simulink model "HVDC_MMC1_EMT"  (R2023b)
settings: Solver=ode23tb  StartTime=0.0  StopTime=10  MaxStep=Ts  RelTol=1e-3  EnableMultiTasking=on
PreLoadFcn:
  | HVDC_MMC_param
StartFcn:
  | tic
StopFcn:
  | toc
values from neighbouring files (symbols this model uses):
  acdcV = 1/(Vnom_dc/2*sqrt(3)/sqrt(2)/Vnom_sec)    [HVDC_MMC_param.m]
  C_PM = 1.758e-3    (= 0.001758)    [HVDC_MMC_param.m]
  Carm = 1.0*C_pm/n    (= 0.0002096)    [B2B_HVDC_MMC_Calc.m]    (also in HVDC_MMC_param.m = 4.88333333333e-05)
  DC_cable_C_shunt = 0.1e-6    (= 1e-07)    [HVDC_MMC_param.m]
  DC_cable_R_shunt = 1000    [HVDC_MMC_param.m]
  DCM = 1    [HVDC_MMC_param.m]
  Fn_filter = 1000    [B2B_HVDC_MMC_Calc.m]    (also in HVDC_MMC_param.m)
  Fnom = 50    [HVDC_MMC_param.m]
  HRM = 2    [HVDC_MMC_param.m]
  HrmOrd = N    (= 2)    [B2B_HVDC_MMC_Calc.m]    (also in HVDC_MMC_param.m)
  Ib_ac = (2/3)*Pnom/Vb_ac    [HVDC_MMC_param.m]
  Ib_dc = Pnom/Vb_dc    (= 1501.5015015)    [HVDC_MMC_param.m]
  Ki_CCSC = 50    [HVDC_MMC_param.m]
  Ki_Ireg = 6    [HVDC_MMC_param.m]
  Ki_Preg = 1.0    (= 1)    [HVDC_MMC_param.m]
  Ki_Qreg = 1.0    (= 1)    [HVDC_MMC_param.m]
  Ki_VDCreg = 100    [HVDC_MMC_param.m]
  Kp_CCSC = 0.8    [HVDC_MMC_param.m]
  Kp_Ireg = 0.6    [HVDC_MMC_param.m]
  Kp_Preg = 0.5/3    (= 0.166666666667)    [HVDC_MMC_param.m]
  Kp_Qreg = 0.5/3    (= 0.166666666667)    [HVDC_MMC_param.m]
  Kp_VDCreg = 4    [HVDC_MMC_param.m]
  L_cable = 15e-3    (= 0.015)    [HVDC_MMC_param.m]
  Larm = Larm_pu*(Zb_ac/w)    [HVDC_MMC_param.m]
  Lff = Larm_pu/2+Lxfo    (= 0.195)    [HVDC_MMC_param.m]
  Limits_Ireg = [ 2.0  -2.0]    [HVDC_MMC_param.m]
  Limits_Preg = [ 1.2, 0.8 ]    [HVDC_MMC_param.m]
  Limits_Qreg = [ 0.25, -0.25 ]    [HVDC_MMC_param.m]
  Limits_VDCreg = [ 2.0  -2.0]    [HVDC_MMC_param.m]
  Lxfo = 0.12    [HVDC_MMC_param.m]
  Pac = 0.9    [HVDC_MMC_param.m]
  Pnom = 1000e6    (= 1000000000)    [HVDC_MMC_param.m]
  Qac = 0.2    [HVDC_MMC_param.m]
  QCM = 0    [HVDC_MMC_param.m]
  R_cable = 0.5    [HVDC_MMC_param.m]
  Rarm = Rarm_pu*Zb_ac    [HVDC_MMC_param.m]
  Rff = Rarm_pu/2+Rxfo    (= 0.00375)    [HVDC_MMC_param.m]
  Rxfo = 0.003    [HVDC_MMC_param.m]
  Slope_Pref = 0.5    [HVDC_MMC_param.m]
  Slope_Qref = 0.5    [HVDC_MMC_param.m]
  Slope_Vdc_ref = Vnom_dc/5    (= 133200)    [HVDC_MMC_param.m]
  Tbrk1_On = 0.1    [HVDC_MMC_param.m]
  Tbrk2_On = 1.0    (= 1)    [HVDC_MMC_param.m]
  Tdeblock = 1.5    [HVDC_MMC_param.m]
  Tfault = 9999    [HVDC_MMC_param.m]
  Ton_Converter2 = 3    [HVDC_MMC_param.m]
  Ton_PQreg = 2    [HVDC_MMC_param.m]
  Ton_VDCreg = 1.5    [HVDC_MMC_param.m]
  Ts = Ts_Power    (= 5e-05)    [B2B_HVDC_MMC_Calc.m]    (also in HVDC_MMC_param.m)
  Ts_Control = Ts_Power    (= 5e-05)    [B2B_HVDC_MMC_Calc.m]    (also in HVDC_MMC_param.m)
  Ts_DQN = MultTs*Ts_Power    (= 5e-05)    [B2B_HVDC_MMC_Calc.m]    (also in HVDC_MMC_param.m)
  Ts_EMT = Ts    (= 5e-05)    [HVDC_MMC_param.m]
  Ts_Power = 1*50e-6    (= 5e-05)    [B2B_HVDC_MMC_Calc.m]    (also in HVDC_MMC_param.m)
  Vb_ac = sqrt(2/3)*Vnom_sec    [HVDC_MMC_param.m]
  Vb_dc = Vnom_dc    (= 666000)    [HVDC_MMC_param.m]
  Vc0_PM = 0    [HVDC_MMC_param.m]
  Vnom_dc = 2*Vnom_sec    (= 666000)    [HVDC_MMC_param.m]
  Vnom_prim = 333e3    (= 333000)    [HVDC_MMC_param.m]
  Vnom_sec = 333e3    (= 333000)    [HVDC_MMC_param.m]
  w = 2*pi*f    (= 314.159265359)    [B2B_HVDC_MMC_Calc.m]    (also in HVDC_MMC_param.m)
  Ws = 2*pi*Fnom    (= 314.159265359)    [HVDC_MMC_param.m]
  Zb_ac = Vb_ac/Ib_ac    [HVDC_MMC_param.m]
  Zeta_filter = 1    [B2B_HVDC_MMC_Calc.m]    (also in HVDC_MMC_param.m)
undefined symbols (not defined in the file or in its folder): DCss, DiscIntNeverNeededParam, gcbh, MT, sps_rtmsupport
libraries: DQN_Lib x37, simulink x35, spsCurrentMeasurementLib x24, powerlib_extras x21, slpidlib x14, spsSecondOrderFilterLib x14, spsVoltageMeasurementLib x10, spsSeriesRLCBranchLib x10, spsControlledVoltageSourceLib x9, spsHalfBridgeMMCmodel x7, spsGroundLib x4, spsParallelRLCBranchLib x4
(part 5 of 9)

== system HVDC_MMC1_EMT/MMC/RHB ==
  Uref : Inport  SampleTime=Ts
  Controlled Voltage Source : spsControlledVoltageSourceLib/Controlled Voltage Source  Initialize=on  Source_Type=AC  Amplitude=0  Phase=0  Frequency=0  Measurements=None
  Controlled Voltage Source2 : spsControlledVoltageSourceLib/Controlled Voltage Source  Initialize=on  Source_Type=AC  Amplitude=0  Phase=0  Frequency=0  Measurements=None
  Current Measurement : spsCurrentMeasurementLib/Current Measurement  PhasorSimulation=off  OutputType=Complex  PSBequivalent=0
  Current Measurement1 : spsCurrentMeasurementLib/Current Measurement  PhasorSimulation=off  OutputType=Complex  PSBequivalent=0
  Demux : Demux  Outputs=2
  Diode : spsDiodeLib/Diode  Ron=Ron_Diode  Lon=0  Vf=Vf_Diode  IC=0  UseSnubber=0  Rs=Rs_Diode  Cs=Cs_Diode  Measurements=off
  Diode1 : spsDiodeLib/Diode  Ron=Ron_Diode  Lon=0  Vf=Vf_Diode  IC=0  UseSnubber=0  Rs=Rs_Diode  Cs=Cs_Diode  Measurements=off
  Discrete-Time Integrator : DiscreteIntegrator  IntegratorMethod=Integration: Trapezoidal  gainval=1  InitialCondition=Vc_Initial  SampleTime=Ts  UpperSaturationLimit=5000  LowerSaturationLimit=500  ICPrevOutput=DiscIntNeverNeededParam  ICPrevScaledInput=DiscIntNeverNeededParam
  Gain : Gain  Gain=1/(C*n)
  Gain2 : Gain  Gain=2
  Mux : Mux  Inputs=2
  Mux1 : Mux  Inputs=2
  Product1 : Product
  Product2 : Product
  Sum1 : Sum  Inputs=1  InputSameDT=on  SaturateOnIntegerOverflow=on  OutDataTypeStr=Inherit: Same as first input
  Sum2 : Sum  Inputs=+-  InputSameDT=on  SaturateOnIntegerOverflow=on  OutDataTypeStr=Inherit: Same as first input
  Unit Delay1 : UnitDelay  SampleTime=Ts  HasFrameUpgradeWarning=on
  Unit Delay3 : UnitDelay  InitialCondition=Vc_Initial  SampleTime=Ts  HasFrameUpgradeWarning=on
  Unit Delay4 : UnitDelay  InitialCondition=Vc_Initial  SampleTime=Ts  HasFrameUpgradeWarning=on
  1 : PMIOPort  Side=Right
  2 : PMIOPort  Port=2  Side=Right
  wires:
  Unit Delay4/1 -> Gain2/1, Unit Delay3/1
  Gain2/1 -> Sum2/1
  Demux/2 -> Controlled Voltage Source2/1
  Sum1/1 -> Gain/1
  Product2/1 -> Demux/1
  Unit Delay3/1 -> Sum2/2
  Mux/1 -> Unit Delay1/1
  Unit Delay1/1 -> Product1/2
  Discrete-Time Integrator/1 -> Unit Delay4/1
  [Icap] -> Mux/2
  Current Measurement1/1 -> [Icap]
  Product1/1 -> Sum1/1
  Current Measurement/1 -> [Imod]
  Mux1/1 -> Product1/1, Product2/1
  Demux/1 -> Controlled Voltage Source/1
  Gain/1 -> Discrete-Time Integrator/1
  Sum2/1 -> Product2/2
  [Imod] -> Mux/1
  Uref/1 -> Mux1/2, Mux1/1
  connections:
  Current Measurement/RConn1 -- Diode1/RConn1 -- Diode/LConn1
  2/RConn1 -- Diode1/LConn1 -- Controlled Voltage Source2/LConn1
  Controlled Voltage Source/RConn1 -- 1/RConn1
  Current Measurement1/RConn1 -- Controlled Voltage Source2/RConn1
  Current Measurement/LConn1 -- Controlled Voltage Source/LConn1
  Diode/RConn1 -- Current Measurement1/LConn1

== system HVDC_MMC1_EMT/MMC/Subsystem ==
  Current Measurement1 : spsCurrentMeasurementLib/Current Measurement  PhasorSimulation=off  OutputType=Complex  PSBequivalent=0
  Voltage Measurement : spsVoltageMeasurementLib/Voltage Measurement  PhasorSimulation=off  OutputType=Complex  PSBequivalent=0
  I1 : PMIOPort  Side=Left
  I2 : PMIOPort  Port=2  Side=Left
  O1 : PMIOPort  Port=3  Side=Right
  O2 : PMIOPort  Port=4  Side=Right
  tag scope: I_Ap=global, V12_Ap=global
  wires:
  Current Measurement1/1 -> [I_Ap]
  Voltage Measurement/1 -> [V12_Ap]
  connections:
  Current Measurement1/RConn1 -- Voltage Measurement/LConn1 -- I1/RConn1
  Current Measurement1/LConn1 -- O1/RConn1
  I2/RConn1 -- Voltage Measurement/LConn2 -- O2/RConn1

== system HVDC_MMC1_EMT/MMC/Subsystem1 ==
  Current Measurement1 : spsCurrentMeasurementLib/Current Measurement  PhasorSimulation=off  OutputType=Complex  PSBequivalent=0
  Voltage Measurement : spsVoltageMeasurementLib/Voltage Measurement  PhasorSimulation=off  OutputType=Complex  PSBequivalent=0
  I1 : PMIOPort  Side=Left
  I2 : PMIOPort  Port=2  Side=Left
  O1 : PMIOPort  Port=3  Side=Right
  O2 : PMIOPort  Port=4  Side=Right
  tag scope: I_Am=global, V12_Am=global
  wires:
  Voltage Measurement/1 -> [V12_Am]
  Current Measurement1/1 -> [I_Am]
  connections:
  Voltage Measurement/LConn2 -- O2/RConn1 -- I2/RConn1
  Current Measurement1/LConn1 -- O1/RConn1
  Voltage Measurement/LConn1 -- Current Measurement1/RConn1 -- I1/RConn1

== system HVDC_MMC1_EMT/MMC/Subsystem2 ==
  Current Measurement1 : spsCurrentMeasurementLib/Current Measurement  PhasorSimulation=off  OutputType=Complex  PSBequivalent=0
  Voltage Measurement : spsVoltageMeasurementLib/Voltage Measurement  PhasorSimulation=off  OutputType=Complex  PSBequivalent=0
  I1 : PMIOPort  Side=Left
  I2 : PMIOPort  Port=2  Side=Left
  O1 : PMIOPort  Port=3  Side=Right
  O2 : PMIOPort  Port=4  Side=Right
  tag scope: I_Bp=global, V12_Bp=global
  wires:
  Voltage Measurement/1 -> [V12_Bp]
  Current Measurement1/1 -> [I_Bp]
  connections:
  Voltage Measurement/LConn2 -- O2/RConn1 -- I2/RConn1
  Current Measurement1/LConn1 -- O1/RConn1
  Voltage Measurement/LConn1 -- Current Measurement1/RConn1 -- I1/RConn1

== system HVDC_MMC1_EMT/MMC/Subsystem3 ==
  Current Measurement1 : spsCurrentMeasurementLib/Current Measurement  PhasorSimulation=off  OutputType=Complex  PSBequivalent=0
  Voltage Measurement : spsVoltageMeasurementLib/Voltage Measurement  PhasorSimulation=off  OutputType=Complex  PSBequivalent=0
  I1 : PMIOPort  Side=Left
  I2 : PMIOPort  Port=2  Side=Left
  O1 : PMIOPort  Port=3  Side=Right
  O2 : PMIOPort  Port=4  Side=Right
  tag scope: I_Bm=global, V12_Bm=global
  wires:
  Current Measurement1/1 -> [I_Bm]
  Voltage Measurement/1 -> [V12_Bm]
  connections:
  I1/RConn1 -- Current Measurement1/RConn1 -- Voltage Measurement/LConn1
  Current Measurement1/LConn1 -- O1/RConn1
  I2/RConn1 -- O2/RConn1 -- Voltage Measurement/LConn2

== system HVDC_MMC1_EMT/MMC/Subsystem4 ==
  Current Measurement1 : spsCurrentMeasurementLib/Current Measurement  PhasorSimulation=off  OutputType=Complex  PSBequivalent=0
  Voltage Measurement : spsVoltageMeasurementLib/Voltage Measurement  PhasorSimulation=off  OutputType=Complex  PSBequivalent=0
  I1 : PMIOPort  Side=Left
  I2 : PMIOPort  Port=2  Side=Left
  O1 : PMIOPort  Port=3  Side=Right
  O2 : PMIOPort  Port=4  Side=Right
  tag scope: I_Cp=global, V12_Cp=global
  wires:
  Current Measurement1/1 -> [I_Cp]
  Voltage Measurement/1 -> [V12_Cp]
  connections:
  I1/RConn1 -- Current Measurement1/RConn1 -- Voltage Measurement/LConn1
  Current Measurement1/LConn1 -- O1/RConn1
  I2/RConn1 -- O2/RConn1 -- Voltage Measurement/LConn2

== system HVDC_MMC1_EMT/MMC/Subsystem5 ==
  Current Measurement1 : spsCurrentMeasurementLib/Current Measurement  PhasorSimulation=off  OutputType=Complex  PSBequivalent=0
  Voltage Measurement : spsVoltageMeasurementLib/Voltage Measurement  PhasorSimulation=off  OutputType=Complex  PSBequivalent=0
  I1 : PMIOPort  Side=Left
  I2 : PMIOPort  Port=2  Side=Left
  O1 : PMIOPort  Port=3  Side=Right
  O2 : PMIOPort  Port=4  Side=Right
  tag scope: I_Cm=global, V12_Cm=global
  wires:
  Voltage Measurement/1 -> [V12_Cm]
  Current Measurement1/1 -> [I_Cm]
  connections:
  Voltage Measurement/LConn2 -- O2/RConn1 -- I2/RConn1
  Current Measurement1/LConn1 -- O1/RConn1
  Voltage Measurement/LConn1 -- Current Measurement1/RConn1 -- I1/RConn1

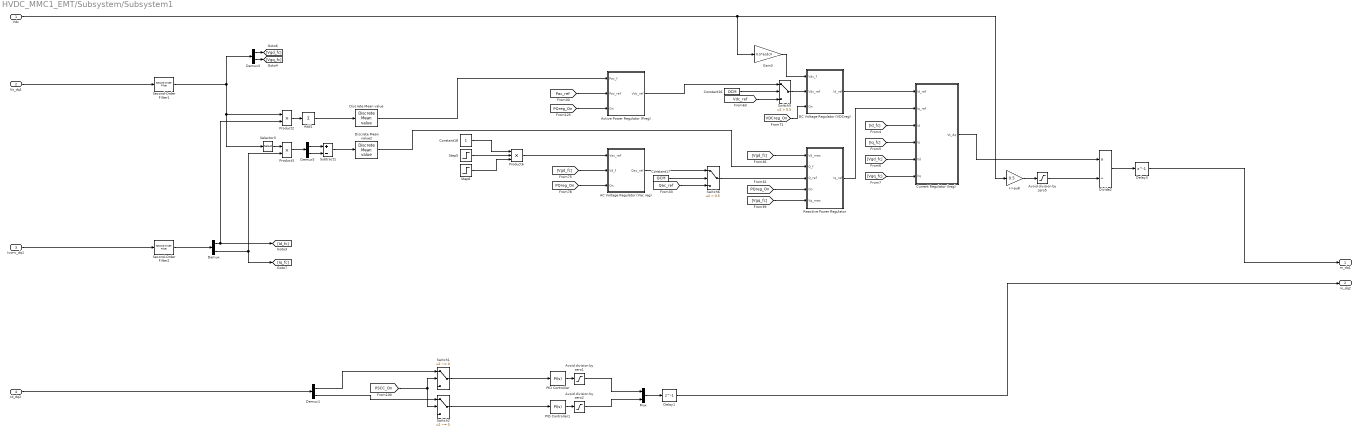
== system HVDC_MMC1_EMT/Subsystem/Subsystem1 ==
  Vdc : Inport
  Vs_dq1 : Inport  Port=2
  Iconv_dq1 : Inport  Port=3
  Id_dq2 : Inport  Port=4
  AC Voltage Regulator (Vac reg) : Subsystem
  Active Power Regulator (Preg) : Subsystem
  Add1 : Sum  Inputs=1
  Avoid division by zero1 : Saturate  UpperLimit=2  LowerLimit=-2
  Avoid division by zero2 : Saturate  UpperLimit=2  LowerLimit=-2
  Avoid division by zero5 : Saturate  UpperLimit=10*acdcV  LowerLimit=0.5/acdcV  ZeroCross=off
  Constant16 : Constant  Value=DCM
  Constant17 : Constant  Value=QCM
  Constant18 : Constant
  Current Regulator (Ireg) : Subsystem
  DC Voltage Regulator (VDCreg) : Subsystem
  Delay1 : Delay  DelayLength=1
  Delay3 : Delay  DelayLength=1
  Demux{,1,3,5} (4 alike) : Demux  Outputs=2
  Discrete Mean value : powerlib_extras/Discrete Measurements/Discrete  Mean value  Freq=Fnom  Vinit=0  Ts=Ts
  Discrete Mean value2 : powerlib_extras/Discrete Measurements/Discrete  Mean value  Freq=Fnom  Vinit=0  Ts=Ts
  Divide2 : Product  Inputs=*/
  Gain3 : Gain  Gain=0.5*acdcV
  I->pu8 : Gain  Gain=0.5  SaturateOnIntegerOverflow=on  OutDataTypeStr=Inherit: Same as input  ParamDataTypeStr=Inherit: Same as input
  Mux : Mux  Inputs=2
  PID Controller : slpidlib/PID Controller  Controller=PI  Form=Parallel  TimeDomain=Continuous-time  UseExternalTs=off  SampleTime=-1  IntegratorMethod=Forward Euler  FilterMethod=Forward Euler  ControllerParametersSource=internal  P=Kp_CCSC  I=Ki_CCSC  UseKiTs=off  D=0  N=100  UseFilter=on  TunerSelectOption=Transfer Function Based (PID Tuner App)  InitialConditionSource=internal  InitialConditionForIntegrator=0  InitialConditionForFilter=0  DifferentiatorICPrevScaledInput=0  ExternalReset=none  TrackingMode=off  Kt=1  LimitOutput=off  SatLimitsSource=internal  UpperSaturationLimit=inf  LowerSaturationLimit=-inf  LinearizeAsGain=on  AntiWindupMode=none  Kb=1  LimitIntegrator=off  UpperIntegratorSaturationLimit=inf  LowerIntegratorSaturationLimit=-inf  POutMin=[]  POutMax=[]  IOutMin=[]  IOutMax=[]  DOutMin=[]  DOutMax=[]  NOutMin=[]  NOutMax=[]  SumOutMin=[]  SumOutMax=[]  SaturationOutMin=[]  SaturationOutMax=[]  PParamMin=[]  PParamMax=[]  IParamMin=[]  IParamMax=[]  DParamMin=[]  DParamMax=[]  NParamMin=[]  NParamMax=[]  KbParamMin=[]  KbParamMax=[]  KtParamMin=[]  KtParamMax=[]  KbOutMin=[]  KbOutMax=[]  KtOutMin=[]  KtOutMax=[]  IntegratorOutMin=[]  IntegratorOutMax=[]  FilterOutMin=[]  FilterOutMax=[]  SumI1OutMin=[]  SumI1OutMax=[]  SumI2OutMin=[]  SumI2OutMax=[]  SumI3OutMin=[]  SumI3OutMax=[]  SumI4OutMin=[]  SumI4OutMax=[]  SumDOutMin=[]  SumDOutMax=[]  DifferentiatorOutMin=[]  DifferentiatorOutMax=[]  FilterDiffOutCoefMin=[]  FilterDiffOutCoefMax=[]  ReciprocalOutMin=[]  ReciprocalOutMax=[]  SumDenOutMin=[]  SumDenOutMax=[]  SumNumOutMin=[]  SumNumOutMax=[]  DivideOutMin=[]  DivideOutMax=[]  UdiffTsProdOutMin=[]  UdiffTsProdOutMax=[]  NTsProdOutMin=[]  NTsProdOutMax=[]  UintegralTsProdOutMin=[]  UintegralTsProdOutMax=[]  UngainTsProdOutMin=[]  UngainTsProdOutMax=[]  ClampingZeroOutDataTypeStr=Inherit: Inherit via back propagation  ClampingZeroOutMin=[]  ClampingZeroOutMax=[]  FilterDenConstantOutDataTypeStr=Inherit: Inherit via back propagation  FilterDenConstantOutMin=[]  FilterDenConstantOutMax=[]  PCopyOutDataTypeStr=Inherit: Inherit via back propagation  PCopyOutMin=[]  PCopyOutMax=[]  NCopyOutDataTypeStr=Inherit: Inherit via back propagation  NCopyOutMin=[]  NCopyOutMax=[]  IntegratorContinuousStateAttributes=''  IntegratorStateMustResolveToSignalObject=off  IntegratorRTWStateStorageClass=Auto  FilterContinuousStateAttributes=''  FilterStateMustResolveToSignalObject=off  FilterRTWStateStorageClass=Auto  ParallelPVariant=InternalParameters  IdealPVariant=Disabled  IVariant=InternalParameters  DVariant=Disabled  IntegratorVariant=Continuous  SatVariant=Disabled  AWVariant=Passthrough  PCopyVariant=Disabled  TRVariant=Disabled  FdbkBlocksVariant=Forward  IdealPFdbkVariant=Disabled  SatFdbkVariant=Disabled  DerivativeFilterVariant=Disabled  NVariant=Disabled  NCopyVariant=Disabled_SignalSpec  FilterICVariant=Disabled  IntegratorICVariant=InternalICs  ExternalResetVariant=Disabled  TRSumVariant=Passthrough  SumFdbkVariant=Disabled  SumVariant=Sum_PI  TsampFilterVariant=InternalTs  TsampNgainVariant=Passthrough  TsampIntegralVariant=Disabled_SignalSpec  ExternalSaturationOutDataTypeStr=Inherit: Same as second input
  PID Controller1 : slpidlib/PID Controller  Controller=PI  Form=Parallel  TimeDomain=Continuous-time  UseExternalTs=off  SampleTime=-1  IntegratorMethod=Forward Euler  FilterMethod=Forward Euler  ControllerParametersSource=internal  P=Kp_CCSC  I=Ki_CCSC  UseKiTs=off  D=0  N=100  UseFilter=on  TunerSelectOption=Transfer Function Based (PID Tuner App)  InitialConditionSource=internal  InitialConditionForIntegrator=0  InitialConditionForFilter=0  DifferentiatorICPrevScaledInput=0  ExternalReset=none  TrackingMode=off  Kt=1  LimitOutput=off  SatLimitsSource=internal  UpperSaturationLimit=inf  LowerSaturationLimit=-inf  LinearizeAsGain=on  AntiWindupMode=none  Kb=1  LimitIntegrator=off  UpperIntegratorSaturationLimit=inf  LowerIntegratorSaturationLimit=-inf  POutMin=[]  POutMax=[]  IOutMin=[]  IOutMax=[]  DOutMin=[]  DOutMax=[]  NOutMin=[]  NOutMax=[]  SumOutMin=[]  SumOutMax=[]  SaturationOutMin=[]  SaturationOutMax=[]  PParamMin=[]  PParamMax=[]  IParamMin=[]  IParamMax=[]  DParamMin=[]  DParamMax=[]  NParamMin=[]  NParamMax=[]  KbParamMin=[]  KbParamMax=[]  KtParamMin=[]  KtParamMax=[]  KbOutMin=[]  KbOutMax=[]  KtOutMin=[]  KtOutMax=[]  IntegratorOutMin=[]  IntegratorOutMax=[]  FilterOutMin=[]  FilterOutMax=[]  SumI1OutMin=[]  SumI1OutMax=[]  SumI2OutMin=[]  SumI2OutMax=[]  SumI3OutMin=[]  SumI3OutMax=[]  SumI4OutMin=[]  SumI4OutMax=[]  SumDOutMin=[]  SumDOutMax=[]  DifferentiatorOutMin=[]  DifferentiatorOutMax=[]  FilterDiffOutCoefMin=[]  FilterDiffOutCoefMax=[]  ReciprocalOutMin=[]  ReciprocalOutMax=[]  SumDenOutMin=[]  SumDenOutMax=[]  SumNumOutMin=[]  SumNumOutMax=[]  DivideOutMin=[]  DivideOutMax=[]  UdiffTsProdOutMin=[]  UdiffTsProdOutMax=[]  NTsProdOutMin=[]  NTsProdOutMax=[]  UintegralTsProdOutMin=[]  UintegralTsProdOutMax=[]  UngainTsProdOutMin=[]  UngainTsProdOutMax=[]  ClampingZeroOutDataTypeStr=Inherit: Inherit via back propagation  ClampingZeroOutMin=[]  ClampingZeroOutMax=[]  FilterDenConstantOutDataTypeStr=Inherit: Inherit via back propagation  FilterDenConstantOutMin=[]  FilterDenConstantOutMax=[]  PCopyOutDataTypeStr=Inherit: Inherit via back propagation  PCopyOutMin=[]  PCopyOutMax=[]  NCopyOutDataTypeStr=Inherit: Inherit via back propagation  NCopyOutMin=[]  NCopyOutMax=[]  IntegratorContinuousStateAttributes=''  IntegratorStateMustResolveToSignalObject=off  IntegratorRTWStateStorageClass=Auto  FilterContinuousStateAttributes=''  FilterStateMustResolveToSignalObject=off  FilterRTWStateStorageClass=Auto  ParallelPVariant=InternalParameters  IdealPVariant=Disabled  IVariant=InternalParameters  DVariant=Disabled  IntegratorVariant=Continuous  SatVariant=Disabled  AWVariant=Passthrough  PCopyVariant=Disabled  TRVariant=Disabled  FdbkBlocksVariant=Forward  IdealPFdbkVariant=Disabled  SatFdbkVariant=Disabled  DerivativeFilterVariant=Disabled  NVariant=Disabled  NCopyVariant=Disabled_SignalSpec  FilterICVariant=Disabled  IntegratorICVariant=InternalICs  ExternalResetVariant=Disabled  TRSumVariant=Passthrough  SumFdbkVariant=Disabled  SumVariant=Sum_PI  TsampFilterVariant=InternalTs  TsampNgainVariant=Passthrough  TsampIntegralVariant=Disabled_SignalSpec  ExternalSaturationOutDataTypeStr=Inherit: Same as second input
  Product2 : Product  RndMeth=Zero
  Product3 : Product  RndMeth=Zero
  Product6 : Product  Inputs=3
  Reactive Power Regulator : Subsystem
  Second-Order Filter1 : spsSecondOrderFilterLib/Second-Order Filter  FilterType=Lowpass  Fo=Fn_filter  Zeta=Zeta_filter  Ts=Ts  Initialize=off  Vac_Init="[0,  0,  60]"  Vdc_Init=0  PlotResponse=off  FreqRange=[0, 500, 1]
  Second-Order Filter2 : spsSecondOrderFilterLib/Second-Order Filter  FilterType=Lowpass  Fo=Fn_filter  Zeta=Zeta_filter  Ts=Ts  Initialize=off  Vac_Init="[0,  0,  60]"  Vdc_Init=0  PlotResponse=off  FreqRange=[0, 500, 1]
  Selector3 : Selector  InputPortWidth=2  IndexOptions=Index vector (dialog)  Indices=[2 1]  OutputSizes=1
  Step5 : Step  Time=7  Before=1  After=0.99  SampleTime=0
  Step6 : Step  Time=9  Before=1  After=1.01/0.99  SampleTime=0
  Subtract1 : Sum  Inputs=+-
  Switch1 : Switch  Criteria=u2 ~= 0  Threshold=0.5  OutDataTypeStr=double  SaturateOnIntegerOverflow=off  InputSameDT=off
  Switch2 : Switch  Criteria=u2 ~= 0  Threshold=0.5  OutDataTypeStr=double  SaturateOnIntegerOverflow=off  InputSameDT=off
  Switch5 : Switch  Criteria=u2 > Threshold  Threshold=0.5  OutDataTypeStr=double  SaturateOnIntegerOverflow=off  InputSameDT=off
  Switch6 : Switch  Criteria=u2 > Threshold  Threshold=0.5  OutDataTypeStr=double  SaturateOnIntegerOverflow=off  InputSameDT=off
  m_dq1 : Outport
  m_dq2 : Outport  Port=2
  wires:
  DC Voltage Regulator (VDCreg)/1(Id_ref) -> Current Regulator (Ireg)/1(Id_ref)
  Second-Order Filter2/1 -> Demux/1
  Demux/2 -> Product3/2, [Iq_fc]
  Switch1/1 -> PID Controller/1
  Active Power Regulator (Preg)/1(Vdc_ref) -> Switch5/1
  [PQreg_On] -> AC Voltage Regulator (Vac reg)/3(On)
  Vdc/1 -> I->pu8/1, Gain3/1
  Avoid division by zero2/1 -> Mux/2
  Mux/1 -> Delay1/1
  Demux3/1 -> [Vgd_fc]
  PID Controller1/1 -> Avoid division by zero2/1
  [Vgq_fc] -> Reactive Power Regulator/5(Vq_mes)
  [Vgq_fc] -> Current Regulator (Ireg)/6(Vq)
  Add1/1 -> Discrete Mean value/1
  Switch6/1 -> Reactive Power Regulator/3(Q_ref)
  Product6/1 -> AC Voltage Regulator (Vac reg)/1(Vac_ref)
  Product2/1 -> Add1/1
  Discrete Mean value/1 -> Active Power Regulator (Preg)/1(Pac_f)
  PID Controller/1 -> Avoid division by zero1/1
  Current Regulator (Ireg)/1(Vt_dq) -> Divide2/1
  Demux5/1 -> Subtract1/1
  [Iq_fc] -> Current Regulator (Ireg)/4(Iq)
  Divide2/1 -> Delay3/1
  I->pu8/1 -> Avoid division by zero5/1
  Constant18/1 -> Product6/1
  [Qac_ref] -> Switch6/3
  Selector3/1 -> Product3/1
  [PQreg_On] -> Reactive Power Regulator/4(On)
  Gain3/1 -> DC Voltage Regulator (VDCreg)/1(Vdc_f)
  Constant17/1 -> Switch6/2
  [Vgd_fc] -> AC Voltage Regulator (Vac reg)/2(Vd_f)
  Demux3/2 -> [Vgq_fc]
  Constant16/1 -> Switch5/2
  Reactive Power Regulator/1(Iq_ref) -> Current Regulator (Ireg)/2(Iq_ref)
  [VDCreg_On] -> DC Voltage Regulator (VDCreg)/3(On)
  Switch5/1 -> DC Voltage Regulator (VDCreg)/2(Vdc_ref)
  [Vgd_fc] -> Reactive Power Regulator/1(Vd_mes)
  [PSCC_On] -> Switch1/2, Switch2/2
  Subtract1/1 -> Discrete Mean value2/1
  Product3/1 -> Demux5/1
  Switch2/1 -> PID Controller1/1
  Avoid division by zero5/1 -> Divide2/2
  Step6/1 -> Product6/3
  Demux5/2 -> Subtract1/2
  AC Voltage Regulator (Vac reg)/1(Qac_ref) -> Switch6/1
  Step5/1 -> Product6/2
  Demux/1 -> [Id_fc], Product2/2
  [Pac_ref] -> Active Power Regulator (Preg)/2(Pac_ref)
  [Id_fc] -> Current Regulator (Ireg)/3(Id)
  Second-Order Filter1/1 -> Selector3/1, Product2/1, Demux3/1
  Avoid division by zero1/1 -> Mux/1
  Iconv_dq1/1 -> Second-Order Filter2/1
  [PQreg_On] -> Active Power Regulator (Preg)/3(On)
  [Vgd_fc] -> Current Regulator (Ireg)/5(Vd)
  Discrete Mean value2/1 -> Reactive Power Regulator/2(Q_f)
  [Vdc_ref] -> Switch5/3
  Delay3/1 -> m_dq1/1
  Delay1/1 -> m_dq2/1
  Vs_dq1/1 -> Second-Order Filter1/1
  Demux1/1 -> Switch1/1
  Demux1/2 -> Switch2/1
  Id_dq2/1 -> Demux1/1

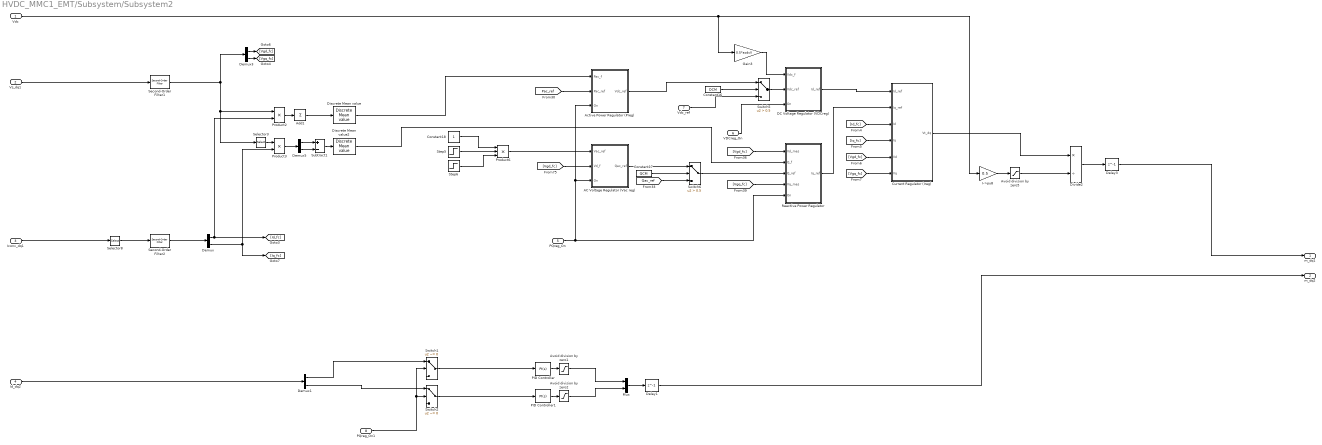
== system HVDC_MMC1_EMT/Subsystem/Subsystem2 ==
  Vdc : Inport
  Vs_dq1 : Inport  Port=2
  Iconv_dq1 : Inport  Port=3
  Id_dq2 : Inport  Port=4
  PQreg_On : Inport  Port=5
  VDCreg_On : Inport  Port=6
  Vdc_ref : Inport  Port=7
  PQreg_On1 : Inport  Port=8
  AC Voltage Regulator (Vac reg) : Subsystem
  Active Power Regulator (Preg) : Subsystem
  Add1 : Sum  Inputs=1
  Avoid division by zero1 : Saturate  UpperLimit=2  LowerLimit=-2
  Avoid division by zero2 : Saturate  UpperLimit=2  LowerLimit=-2
  Avoid division by zero5 : Saturate  UpperLimit=10*acdcV  LowerLimit=0.5/acdcV  ZeroCross=off
  Constant16 : Constant  Value=DCM
  Constant17 : Constant  Value=QCM
  Constant18 : Constant
  Current Regulator (Ireg) : Subsystem
  DC Voltage Regulator (VDCreg) : Subsystem
  Delay1 : Delay  DelayLength=1
  Delay3 : Delay  DelayLength=1
  Demux{,1,3,5} (4 alike) : Demux  Outputs=2
  Discrete Mean value : powerlib_extras/Discrete Measurements/Discrete  Mean value  Freq=Fnom  Vinit=0  Ts=Ts
  Discrete Mean value2 : powerlib_extras/Discrete Measurements/Discrete  Mean value  Freq=Fnom  Vinit=0  Ts=Ts
  Divide2 : Product  Inputs=*/
  Gain3 : Gain  Gain=0.5*acdcV
  I->pu8 : Gain  Gain=0.5  SaturateOnIntegerOverflow=on  OutDataTypeStr=Inherit: Same as input  ParamDataTypeStr=Inherit: Same as input
  Mux : Mux  Inputs=2
  PID Controller : slpidlib/PID Controller  Controller=PI  Form=Parallel  TimeDomain=Continuous-time  UseExternalTs=off  SampleTime=-1  IntegratorMethod=Forward Euler  FilterMethod=Forward Euler  ControllerParametersSource=internal  P=Kp_CCSC  I=Ki_CCSC  UseKiTs=off  D=0  N=100  UseFilter=on  TunerSelectOption=Transfer Function Based (PID Tuner App)  InitialConditionSource=internal  InitialConditionForIntegrator=0  InitialConditionForFilter=0  DifferentiatorICPrevScaledInput=0  ExternalReset=none  TrackingMode=off  Kt=1  LimitOutput=off  SatLimitsSource=internal  UpperSaturationLimit=inf  LowerSaturationLimit=-inf  LinearizeAsGain=on  AntiWindupMode=none  Kb=1  LimitIntegrator=off  UpperIntegratorSaturationLimit=inf  LowerIntegratorSaturationLimit=-inf  POutMin=[]  POutMax=[]  IOutMin=[]  IOutMax=[]  DOutMin=[]  DOutMax=[]  NOutMin=[]  NOutMax=[]  SumOutMin=[]  SumOutMax=[]  SaturationOutMin=[]  SaturationOutMax=[]  PParamMin=[]  PParamMax=[]  IParamMin=[]  IParamMax=[]  DParamMin=[]  DParamMax=[]  NParamMin=[]  NParamMax=[]  KbParamMin=[]  KbParamMax=[]  KtParamMin=[]  KtParamMax=[]  KbOutMin=[]  KbOutMax=[]  KtOutMin=[]  KtOutMax=[]  IntegratorOutMin=[]  IntegratorOutMax=[]  FilterOutMin=[]  FilterOutMax=[]  SumI1OutMin=[]  SumI1OutMax=[]  SumI2OutMin=[]  SumI2OutMax=[]  SumI3OutMin=[]  SumI3OutMax=[]  SumI4OutMin=[]  SumI4OutMax=[]  SumDOutMin=[]  SumDOutMax=[]  DifferentiatorOutMin=[]  DifferentiatorOutMax=[]  FilterDiffOutCoefMin=[]  FilterDiffOutCoefMax=[]  ReciprocalOutMin=[]  ReciprocalOutMax=[]  SumDenOutMin=[]  SumDenOutMax=[]  SumNumOutMin=[]  SumNumOutMax=[]  DivideOutMin=[]  DivideOutMax=[]  UdiffTsProdOutMin=[]  UdiffTsProdOutMax=[]  NTsProdOutMin=[]  NTsProdOutMax=[]  UintegralTsProdOutMin=[]  UintegralTsProdOutMax=[]  UngainTsProdOutMin=[]  UngainTsProdOutMax=[]  ClampingZeroOutDataTypeStr=Inherit: Inherit via back propagation  ClampingZeroOutMin=[]  ClampingZeroOutMax=[]  FilterDenConstantOutDataTypeStr=Inherit: Inherit via back propagation  FilterDenConstantOutMin=[]  FilterDenConstantOutMax=[]  PCopyOutDataTypeStr=Inherit: Inherit via back propagation  PCopyOutMin=[]  PCopyOutMax=[]  NCopyOutDataTypeStr=Inherit: Inherit via back propagation  NCopyOutMin=[]  NCopyOutMax=[]  IntegratorContinuousStateAttributes=''  IntegratorStateMustResolveToSignalObject=off  IntegratorRTWStateStorageClass=Auto  FilterContinuousStateAttributes=''  FilterStateMustResolveToSignalObject=off  FilterRTWStateStorageClass=Auto  ParallelPVariant=InternalParameters  IdealPVariant=Disabled  IVariant=InternalParameters  DVariant=Disabled  IntegratorVariant=Continuous  SatVariant=Disabled  AWVariant=Passthrough  PCopyVariant=Disabled  TRVariant=Disabled  FdbkBlocksVariant=Forward  IdealPFdbkVariant=Disabled  SatFdbkVariant=Disabled  DerivativeFilterVariant=Disabled  NVariant=Disabled  NCopyVariant=Disabled_SignalSpec  FilterICVariant=Disabled  IntegratorICVariant=InternalICs  ExternalResetVariant=Disabled  TRSumVariant=Passthrough  SumFdbkVariant=Disabled  SumVariant=Sum_PI  TsampFilterVariant=InternalTs  TsampNgainVariant=Passthrough  TsampIntegralVariant=Disabled_SignalSpec  ExternalSaturationOutDataTypeStr=Inherit: Same as second input
  PID Controller1 : slpidlib/PID Controller  Controller=PI  Form=Parallel  TimeDomain=Continuous-time  UseExternalTs=off  SampleTime=-1  IntegratorMethod=Forward Euler  FilterMethod=Forward Euler  ControllerParametersSource=internal  P=Kp_CCSC  I=Ki_CCSC  UseKiTs=off  D=0  N=100  UseFilter=on  TunerSelectOption=Transfer Function Based (PID Tuner App)  InitialConditionSource=internal  InitialConditionForIntegrator=0  InitialConditionForFilter=0  DifferentiatorICPrevScaledInput=0  ExternalReset=none  TrackingMode=off  Kt=1  LimitOutput=off  SatLimitsSource=internal  UpperSaturationLimit=inf  LowerSaturationLimit=-inf  LinearizeAsGain=on  AntiWindupMode=none  Kb=1  LimitIntegrator=off  UpperIntegratorSaturationLimit=inf  LowerIntegratorSaturationLimit=-inf  POutMin=[]  POutMax=[]  IOutMin=[]  IOutMax=[]  DOutMin=[]  DOutMax=[]  NOutMin=[]  NOutMax=[]  SumOutMin=[]  SumOutMax=[]  SaturationOutMin=[]  SaturationOutMax=[]  PParamMin=[]  PParamMax=[]  IParamMin=[]  IParamMax=[]  DParamMin=[]  DParamMax=[]  NParamMin=[]  NParamMax=[]  KbParamMin=[]  KbParamMax=[]  KtParamMin=[]  KtParamMax=[]  KbOutMin=[]  KbOutMax=[]  KtOutMin=[]  KtOutMax=[]  IntegratorOutMin=[]  IntegratorOutMax=[]  FilterOutMin=[]  FilterOutMax=[]  SumI1OutMin=[]  SumI1OutMax=[]  SumI2OutMin=[]  SumI2OutMax=[]  SumI3OutMin=[]  SumI3OutMax=[]  SumI4OutMin=[]  SumI4OutMax=[]  SumDOutMin=[]  SumDOutMax=[]  DifferentiatorOutMin=[]  DifferentiatorOutMax=[]  FilterDiffOutCoefMin=[]  FilterDiffOutCoefMax=[]  ReciprocalOutMin=[]  ReciprocalOutMax=[]  SumDenOutMin=[]  SumDenOutMax=[]  SumNumOutMin=[]  SumNumOutMax=[]  DivideOutMin=[]  DivideOutMax=[]  UdiffTsProdOutMin=[]  UdiffTsProdOutMax=[]  NTsProdOutMin=[]  NTsProdOutMax=[]  UintegralTsProdOutMin=[]  UintegralTsProdOutMax=[]  UngainTsProdOutMin=[]  UngainTsProdOutMax=[]  ClampingZeroOutDataTypeStr=Inherit: Inherit via back propagation  ClampingZeroOutMin=[]  ClampingZeroOutMax=[]  FilterDenConstantOutDataTypeStr=Inherit: Inherit via back propagation  FilterDenConstantOutMin=[]  FilterDenConstantOutMax=[]  PCopyOutDataTypeStr=Inherit: Inherit via back propagation  PCopyOutMin=[]  PCopyOutMax=[]  NCopyOutDataTypeStr=Inherit: Inherit via back propagation  NCopyOutMin=[]  NCopyOutMax=[]  IntegratorContinuousStateAttributes=''  IntegratorStateMustResolveToSignalObject=off  IntegratorRTWStateStorageClass=Auto  FilterContinuousStateAttributes=''  FilterStateMustResolveToSignalObject=off  FilterRTWStateStorageClass=Auto  ParallelPVariant=InternalParameters  IdealPVariant=Disabled  IVariant=InternalParameters  DVariant=Disabled  IntegratorVariant=Continuous  SatVariant=Disabled  AWVariant=Passthrough  PCopyVariant=Disabled  TRVariant=Disabled  FdbkBlocksVariant=Forward  IdealPFdbkVariant=Disabled  SatFdbkVariant=Disabled  DerivativeFilterVariant=Disabled  NVariant=Disabled  NCopyVariant=Disabled_SignalSpec  FilterICVariant=Disabled  IntegratorICVariant=InternalICs  ExternalResetVariant=Disabled  TRSumVariant=Passthrough  SumFdbkVariant=Disabled  SumVariant=Sum_PI  TsampFilterVariant=InternalTs  TsampNgainVariant=Passthrough  TsampIntegralVariant=Disabled_SignalSpec  ExternalSaturationOutDataTypeStr=Inherit: Same as second input
  Product2 : Product  RndMeth=Zero
  Product3 : Product  RndMeth=Zero
  Product6 : Product  Inputs=3
  Reactive Power Regulator : Subsystem
  Second-Order Filter1 : spsSecondOrderFilterLib/Second-Order Filter  FilterType=Lowpass  Fo=Fn_filter  Zeta=Zeta_filter  Ts=Ts  Initialize=off  Vac_Init="[0,  0,  60]"  Vdc_Init=0  PlotResponse=off  FreqRange=[0, 500, 1]
  Second-Order Filter2 : spsSecondOrderFilterLib/Second-Order Filter  FilterType=Lowpass  Fo=Fn_filter  Zeta=Zeta_filter  Ts=Ts  Initialize=off  Vac_Init="[0,  0,  60]"  Vdc_Init=0  PlotResponse=off  FreqRange=[0, 500, 1]
  Selector3 : Selector  InputPortWidth=2  IndexOptions=Index vector (dialog)  Indices=[2 1]  OutputSizes=1
  Selector8 : Selector  InputPortWidth=2  IndexOptions=Index vector (dialog)  Indices=[1 2]  OutputSizes=1
  Step5 : Step  Time=4.5  Before=1  After=0.99  SampleTime=0
  Step6 : Step  Time=6  Before=1  After=1.01/0.99  SampleTime=0
  Subtract1 : Sum  Inputs=+-
  Switch1 : Switch  Criteria=u2 ~= 0  Threshold=0.5  OutDataTypeStr=double  SaturateOnIntegerOverflow=off  InputSameDT=off
  Switch2 : Switch  Criteria=u2 ~= 0  Threshold=0.5  OutDataTypeStr=double  SaturateOnIntegerOverflow=off  InputSameDT=off
  Switch5 : Switch  Criteria=u2 > Threshold  Threshold=0.5  OutDataTypeStr=double  SaturateOnIntegerOverflow=off  InputSameDT=off
  Switch6 : Switch  Criteria=u2 > Threshold  Threshold=0.5  OutDataTypeStr=double  SaturateOnIntegerOverflow=off  InputSameDT=off
  m_dq1 : Outport
  m_dq2 : Outport  Port=2
  wires:
  DC Voltage Regulator (VDCreg)/1(Id_ref) -> Current Regulator (Ireg)/1(Id_ref)
  Second-Order Filter2/1 -> Demux/1
  Demux/2 -> Product3/2, [Iq_fc]
  Switch1/1 -> PID Controller/1
  Active Power Regulator (Preg)/1(Vdc_ref) -> Switch5/1
  Vdc/1 -> I->pu8/1, Gain3/1
  Avoid division by zero2/1 -> Mux/2
  Mux/1 -> Delay1/1
  Demux3/1 -> [Vgd_fc]
  PID Controller1/1 -> Avoid division by zero2/1
  [Vgq_fc] -> Reactive Power Regulator/4(Vq_mes)
  [Vgq_fc] -> Current Regulator (Ireg)/6(Vq)
  Add1/1 -> Discrete Mean value/1
  Switch6/1 -> Reactive Power Regulator/3(Q_ref)
  Product6/1 -> AC Voltage Regulator (Vac reg)/1(Vac_ref)
  Product2/1 -> Add1/1
  Discrete Mean value/1 -> Active Power Regulator (Preg)/1(Pac_f)
  PID Controller/1 -> Avoid division by zero1/1
  Current Regulator (Ireg)/1(Vt_dq) -> Divide2/1
  Demux5/1 -> Subtract1/1
  [Iq_fc] -> Current Regulator (Ireg)/4(Iq)
  Divide2/1 -> Delay3/1
  I->pu8/1 -> Avoid division by zero5/1
  Constant18/1 -> Product6/1
  [Qac_ref] -> Switch6/3
  Selector3/1 -> Product3/1
  PQreg_On/1 -> AC Voltage Regulator (Vac reg)/3(On), Active Power Regulator (Preg)/3(On), Reactive Power Regulator/5(On)
  Gain3/1 -> DC Voltage Regulator (VDCreg)/1(Vdc_f)
  Constant17/1 -> Switch6/2
  [Vgd_fc] -> AC Voltage Regulator (Vac reg)/2(Vd_f)
  Demux3/2 -> [Vgq_fc]
  Constant16/1 -> Switch5/2
  Reactive Power Regulator/1(Iq_ref) -> Current Regulator (Ireg)/2(Iq_ref)
  Switch5/1 -> DC Voltage Regulator (VDCreg)/2(Vdc_ref)
  [Vgd_fc] -> Reactive Power Regulator/1(Vd_mes)
  PQreg_On1/1 -> Switch1/2, Switch2/2
  Subtract1/1 -> Discrete Mean value2/1
  Product3/1 -> Demux5/1
  Switch2/1 -> PID Controller1/1
  Avoid division by zero5/1 -> Divide2/2
  Step6/1 -> Product6/3
  Demux5/2 -> Subtract1/2
  AC Voltage Regulator (Vac reg)/1(Qac_ref) -> Switch6/1
  Step5/1 -> Product6/2
  Demux/1 -> [Id_fc], Product2/2
  [Pac_ref] -> Active Power Regulator (Preg)/2(Pac_ref)
  [Id_fc] -> Current Regulator (Ireg)/3(Id)
  Second-Order Filter1/1 -> Selector3/1, Product2/1, Demux3/1
  Avoid division by zero1/1 -> Mux/1
  Selector8/1 -> Second-Order Filter2/1
  [Vgd_fc] -> Current Regulator (Ireg)/5(Vd)
  Discrete Mean value2/1 -> Reactive Power Regulator/2(Q_f)
  Vdc_ref/1 -> Switch5/3
  Delay3/1 -> m_dq1/1
  Delay1/1 -> m_dq2/1
  Vs_dq1/1 -> Second-Order Filter1/1
  Iconv_dq1/1 -> Selector8/1
  Demux1/1 -> Switch1/1
  Demux1/2 -> Switch2/1
  Id_dq2/1 -> Demux1/1
  VDCreg_On/1 -> DC Voltage Regulator (VDCreg)/3(On)

== system HVDC_MMC1_EMT/Subsystem1/DC Voltage Regulator (VDCreg)1 ==
  note: VDC Regulator
  Ref : Inport  PortDimensions=1
  Meas : Inport  Port=2  PortDimensions=1
  On : Inport  Port=3  PortDimensions=1
  Discrete-Time Integrator : DiscreteIntegrator  InitialCondition=1  SampleTime=Ts  LimitOutput=on  UpperSaturationLimit=Limits_VDCreg(1)*5  LowerSaturationLimit=Limits_VDCreg(2)*5  ICPrevOutput=DiscIntNeverNeededParam  ICPrevScaledInput=DiscIntNeverNeededParam
  Gain : Gain
  Gain1 : Gain
  Product : Product  RndMeth=Zero
  Product1 : Product  RndMeth=Zero
  Saturation2 : Saturate  UpperLimit=1.5  LowerLimit=0.5  SampleTime=Ts
  Sum : Sum  Inputs=|+-
  Sum6 : Sum  InputSameDT=on  SaturateOnIntegerOverflow=on  SampleTime=Ts  OutDataTypeStr=Inherit: Same as first input
  Switch1 : Switch  Criteria=u2 ~= 0  Threshold=0.5  OutDataTypeStr=double  SaturateOnIntegerOverflow=off  InputSameDT=off
  VdcNom_SM : Constant  Value=0.1
  VdcNom_SM1 : Constant  Value=0.5
  Zero-Order Hold : ZeroOrderHold  SampleTime=Ts
  Id_ref : Outport  VectorParamsAs1DForOutWhenUnconnected=off
  wires:
  Product/1 -> Discrete-Time Integrator/1
  Product1/1 -> Zero-Order Hold/1
  Discrete-Time Integrator/1 -> Sum6/2
  Zero-Order Hold/1 -> Sum6/1
  On/1 -> Switch1/2
  Ref/1 -> Switch1/1
  Sum/1 -> Product/2, Product1/2
  Meas/1 -> Sum/2, Switch1/3
  Switch1/1 -> Sum/1
  VdcNom_SM/1 -> Gain/1
  VdcNom_SM1/1 -> Gain1/1
  Sum6/1 -> Saturation2/1
  Gain/1 -> Product1/1
  Gain1/1 -> Product/1
  Saturation2/1 -> Id_ref/1

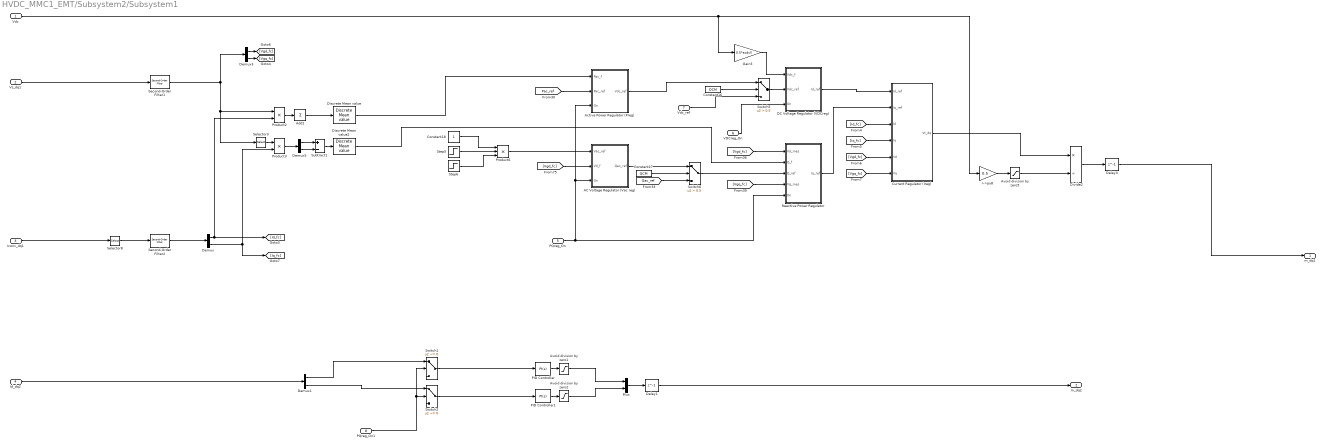
== system HVDC_MMC1_EMT/Subsystem2/Subsystem1 ==
  Vdc : Inport
  Vs_dq1 : Inport  Port=2
  Iconv_dq1 : Inport  Port=3
  Id_dq2 : Inport  Port=4
  PQreg_On : Inport  Port=5
  VDCreg_On : Inport  Port=6
  Vdc_ref : Inport  Port=7
  PQreg_On1 : Inport  Port=8
  AC Voltage Regulator (Vac reg) : Subsystem
  Active Power Regulator (Preg) : Subsystem
  Add1 : Sum  Inputs=1
  Avoid division by zero1 : Saturate  UpperLimit=2  LowerLimit=-2
  Avoid division by zero2 : Saturate  UpperLimit=2  LowerLimit=-2
  Avoid division by zero5 : Saturate  UpperLimit=10*acdcV  LowerLimit=0.5/acdcV  ZeroCross=off
  Constant16 : Constant  Value=DCM
  Constant17 : Constant  Value=QCM
  Constant18 : Constant
  Current Regulator (Ireg) : Subsystem
  DC Voltage Regulator (VDCreg) : Subsystem
  Delay1 : Delay  DelayLength=1
  Delay3 : Delay  DelayLength=1
  Demux{,1,3,5} (4 alike) : Demux  Outputs=2
  Discrete Mean value : powerlib_extras/Discrete Measurements/Discrete  Mean value  Freq=Fnom  Vinit=0  Ts=Ts
  Discrete Mean value2 : powerlib_extras/Discrete Measurements/Discrete  Mean value  Freq=Fnom  Vinit=0  Ts=Ts
  Divide2 : Product  Inputs=*/
  Gain3 : Gain  Gain=0.5*acdcV
  I->pu8 : Gain  Gain=0.5  SaturateOnIntegerOverflow=on  OutDataTypeStr=Inherit: Same as input  ParamDataTypeStr=Inherit: Same as input
  Mux : Mux  Inputs=2
  PID Controller : slpidlib/PID Controller  Controller=PI  Form=Parallel  TimeDomain=Continuous-time  UseExternalTs=off  SampleTime=-1  IntegratorMethod=Forward Euler  FilterMethod=Forward Euler  ControllerParametersSource=internal  P=Kp_CCSC  I=Ki_CCSC  UseKiTs=off  D=0  N=100  UseFilter=on  TunerSelectOption=Transfer Function Based (PID Tuner App)  InitialConditionSource=internal  InitialConditionForIntegrator=0  InitialConditionForFilter=0  DifferentiatorICPrevScaledInput=0  ExternalReset=none  TrackingMode=off  Kt=1  LimitOutput=off  SatLimitsSource=internal  UpperSaturationLimit=inf  LowerSaturationLimit=-inf  LinearizeAsGain=on  AntiWindupMode=none  Kb=1  LimitIntegrator=off  UpperIntegratorSaturationLimit=inf  LowerIntegratorSaturationLimit=-inf  POutMin=[]  POutMax=[]  IOutMin=[]  IOutMax=[]  DOutMin=[]  DOutMax=[]  NOutMin=[]  NOutMax=[]  SumOutMin=[]  SumOutMax=[]  SaturationOutMin=[]  SaturationOutMax=[]  PParamMin=[]  PParamMax=[]  IParamMin=[]  IParamMax=[]  DParamMin=[]  DParamMax=[]  NParamMin=[]  NParamMax=[]  KbParamMin=[]  KbParamMax=[]  KtParamMin=[]  KtParamMax=[]  KbOutMin=[]  KbOutMax=[]  KtOutMin=[]  KtOutMax=[]  IntegratorOutMin=[]  IntegratorOutMax=[]  FilterOutMin=[]  FilterOutMax=[]  SumI1OutMin=[]  SumI1OutMax=[]  SumI2OutMin=[]  SumI2OutMax=[]  SumI3OutMin=[]  SumI3OutMax=[]  SumI4OutMin=[]  SumI4OutMax=[]  SumDOutMin=[]  SumDOutMax=[]  DifferentiatorOutMin=[]  DifferentiatorOutMax=[]  FilterDiffOutCoefMin=[]  FilterDiffOutCoefMax=[]  ReciprocalOutMin=[]  ReciprocalOutMax=[]  SumDenOutMin=[]  SumDenOutMax=[]  SumNumOutMin=[]  SumNumOutMax=[]  DivideOutMin=[]  DivideOutMax=[]  UdiffTsProdOutMin=[]  UdiffTsProdOutMax=[]  NTsProdOutMin=[]  NTsProdOutMax=[]  UintegralTsProdOutMin=[]  UintegralTsProdOutMax=[]  UngainTsProdOutMin=[]  UngainTsProdOutMax=[]  ClampingZeroOutDataTypeStr=Inherit: Inherit via back propagation  ClampingZeroOutMin=[]  ClampingZeroOutMax=[]  FilterDenConstantOutDataTypeStr=Inherit: Inherit via back propagation  FilterDenConstantOutMin=[]  FilterDenConstantOutMax=[]  PCopyOutDataTypeStr=Inherit: Inherit via back propagation  PCopyOutMin=[]  PCopyOutMax=[]  NCopyOutDataTypeStr=Inherit: Inherit via back propagation  NCopyOutMin=[]  NCopyOutMax=[]  IntegratorContinuousStateAttributes=''  IntegratorStateMustResolveToSignalObject=off  IntegratorRTWStateStorageClass=Auto  FilterContinuousStateAttributes=''  FilterStateMustResolveToSignalObject=off  FilterRTWStateStorageClass=Auto  ParallelPVariant=InternalParameters  IdealPVariant=Disabled  IVariant=InternalParameters  DVariant=Disabled  IntegratorVariant=Continuous  SatVariant=Disabled  AWVariant=Passthrough  PCopyVariant=Disabled  TRVariant=Disabled  FdbkBlocksVariant=Forward  IdealPFdbkVariant=Disabled  SatFdbkVariant=Disabled  DerivativeFilterVariant=Disabled  NVariant=Disabled  NCopyVariant=Disabled_SignalSpec  FilterICVariant=Disabled  IntegratorICVariant=InternalICs  ExternalResetVariant=Disabled  TRSumVariant=Passthrough  SumFdbkVariant=Disabled  SumVariant=Sum_PI  TsampFilterVariant=InternalTs  TsampNgainVariant=Passthrough  TsampIntegralVariant=Disabled_SignalSpec  ExternalSaturationOutDataTypeStr=Inherit: Same as second input
  PID Controller1 : slpidlib/PID Controller  Controller=PI  Form=Parallel  TimeDomain=Continuous-time  UseExternalTs=off  SampleTime=-1  IntegratorMethod=Forward Euler  FilterMethod=Forward Euler  ControllerParametersSource=internal  P=Kp_CCSC  I=Ki_CCSC  UseKiTs=off  D=0  N=100  UseFilter=on  TunerSelectOption=Transfer Function Based (PID Tuner App)  InitialConditionSource=internal  InitialConditionForIntegrator=0  InitialConditionForFilter=0  DifferentiatorICPrevScaledInput=0  ExternalReset=none  TrackingMode=off  Kt=1  LimitOutput=off  SatLimitsSource=internal  UpperSaturationLimit=inf  LowerSaturationLimit=-inf  LinearizeAsGain=on  AntiWindupMode=none  Kb=1  LimitIntegrator=off  UpperIntegratorSaturationLimit=inf  LowerIntegratorSaturationLimit=-inf  POutMin=[]  POutMax=[]  IOutMin=[]  IOutMax=[]  DOutMin=[]  DOutMax=[]  NOutMin=[]  NOutMax=[]  SumOutMin=[]  SumOutMax=[]  SaturationOutMin=[]  SaturationOutMax=[]  PParamMin=[]  PParamMax=[]  IParamMin=[]  IParamMax=[]  DParamMin=[]  DParamMax=[]  NParamMin=[]  NParamMax=[]  KbParamMin=[]  KbParamMax=[]  KtParamMin=[]  KtParamMax=[]  KbOutMin=[]  KbOutMax=[]  KtOutMin=[]  KtOutMax=[]  IntegratorOutMin=[]  IntegratorOutMax=[]  FilterOutMin=[]  FilterOutMax=[]  SumI1OutMin=[]  SumI1OutMax=[]  SumI2OutMin=[]  SumI2OutMax=[]  SumI3OutMin=[]  SumI3OutMax=[]  SumI4OutMin=[]  SumI4OutMax=[]  SumDOutMin=[]  SumDOutMax=[]  DifferentiatorOutMin=[]  DifferentiatorOutMax=[]  FilterDiffOutCoefMin=[]  FilterDiffOutCoefMax=[]  ReciprocalOutMin=[]  ReciprocalOutMax=[]  SumDenOutMin=[]  SumDenOutMax=[]  SumNumOutMin=[]  SumNumOutMax=[]  DivideOutMin=[]  DivideOutMax=[]  UdiffTsProdOutMin=[]  UdiffTsProdOutMax=[]  NTsProdOutMin=[]  NTsProdOutMax=[]  UintegralTsProdOutMin=[]  UintegralTsProdOutMax=[]  UngainTsProdOutMin=[]  UngainTsProdOutMax=[]  ClampingZeroOutDataTypeStr=Inherit: Inherit via back propagation  ClampingZeroOutMin=[]  ClampingZeroOutMax=[]  FilterDenConstantOutDataTypeStr=Inherit: Inherit via back propagation  FilterDenConstantOutMin=[]  FilterDenConstantOutMax=[]  PCopyOutDataTypeStr=Inherit: Inherit via back propagation  PCopyOutMin=[]  PCopyOutMax=[]  NCopyOutDataTypeStr=Inherit: Inherit via back propagation  NCopyOutMin=[]  NCopyOutMax=[]  IntegratorContinuousStateAttributes=''  IntegratorStateMustResolveToSignalObject=off  IntegratorRTWStateStorageClass=Auto  FilterContinuousStateAttributes=''  FilterStateMustResolveToSignalObject=off  FilterRTWStateStorageClass=Auto  ParallelPVariant=InternalParameters  IdealPVariant=Disabled  IVariant=InternalParameters  DVariant=Disabled  IntegratorVariant=Continuous  SatVariant=Disabled  AWVariant=Passthrough  PCopyVariant=Disabled  TRVariant=Disabled  FdbkBlocksVariant=Forward  IdealPFdbkVariant=Disabled  SatFdbkVariant=Disabled  DerivativeFilterVariant=Disabled  NVariant=Disabled  NCopyVariant=Disabled_SignalSpec  FilterICVariant=Disabled  IntegratorICVariant=InternalICs  ExternalResetVariant=Disabled  TRSumVariant=Passthrough  SumFdbkVariant=Disabled  SumVariant=Sum_PI  TsampFilterVariant=InternalTs  TsampNgainVariant=Passthrough  TsampIntegralVariant=Disabled_SignalSpec  ExternalSaturationOutDataTypeStr=Inherit: Same as second input
  Product2 : Product  RndMeth=Zero
  Product3 : Product  RndMeth=Zero
  Product6 : Product  Inputs=3
  Reactive Power Regulator : Subsystem
  Second-Order Filter1 : spsSecondOrderFilterLib/Second-Order Filter  FilterType=Lowpass  Fo=Fn_filter  Zeta=Zeta_filter  Ts=Ts  Initialize=off  Vac_Init="[0,  0,  60]"  Vdc_Init=0  PlotResponse=off  FreqRange=[0, 500, 1]
  Second-Order Filter2 : spsSecondOrderFilterLib/Second-Order Filter  FilterType=Lowpass  Fo=Fn_filter  Zeta=Zeta_filter  Ts=Ts  Initialize=off  Vac_Init="[0,  0,  60]"  Vdc_Init=0  PlotResponse=off  FreqRange=[0, 500, 1]
  Selector3 : Selector  InputPortWidth=2  IndexOptions=Index vector (dialog)  Indices=[2 1]  OutputSizes=1
  Selector8 : Selector  InputPortWidth=2  IndexOptions=Index vector (dialog)  Indices=[1 2]  OutputSizes=1
  Step5 : Step  Time=4.5  Before=1  After=0.99  SampleTime=0
  Step6 : Step  Time=6  Before=1  After=1.01/0.99  SampleTime=0
  Subtract1 : Sum  Inputs=+-
  Switch1 : Switch  Criteria=u2 ~= 0  Threshold=0.5  OutDataTypeStr=double  SaturateOnIntegerOverflow=off  InputSameDT=off
  Switch2 : Switch  Criteria=u2 ~= 0  Threshold=0.5  OutDataTypeStr=double  SaturateOnIntegerOverflow=off  InputSameDT=off
  Switch5 : Switch  Criteria=u2 > Threshold  Threshold=0.5  OutDataTypeStr=double  SaturateOnIntegerOverflow=off  InputSameDT=off
  Switch6 : Switch  Criteria=u2 > Threshold  Threshold=0.5  OutDataTypeStr=double  SaturateOnIntegerOverflow=off  InputSameDT=off
  m_dq1 : Outport
  m_dq2 : Outport  Port=2
  wires:
  DC Voltage Regulator (VDCreg)/1(Id_ref) -> Current Regulator (Ireg)/1(Id_ref)
  Second-Order Filter2/1 -> Demux/1
  Demux/2 -> Product3/2, [Iq_fc]
  Switch1/1 -> PID Controller/1
  Active Power Regulator (Preg)/1(Vdc_ref) -> Switch5/1
  Vdc/1 -> I->pu8/1, Gain3/1
  Avoid division by zero2/1 -> Mux/2
  Mux/1 -> Delay1/1
  Demux3/1 -> [Vgd_fc]
  PID Controller1/1 -> Avoid division by zero2/1
  [Vgq_fc] -> Reactive Power Regulator/4(Vq_mes)
  [Vgq_fc] -> Current Regulator (Ireg)/6(Vq)
  Add1/1 -> Discrete Mean value/1
  Switch6/1 -> Reactive Power Regulator/3(Q_ref)
  Product6/1 -> AC Voltage Regulator (Vac reg)/1(Vac_ref)
  Product2/1 -> Add1/1
  Discrete Mean value/1 -> Active Power Regulator (Preg)/1(Pac_f)
  PID Controller/1 -> Avoid division by zero1/1
  Current Regulator (Ireg)/1(Vt_dq) -> Divide2/1
  Demux5/1 -> Subtract1/1
  [Iq_fc] -> Current Regulator (Ireg)/4(Iq)
  Divide2/1 -> Delay3/1
  I->pu8/1 -> Avoid division by zero5/1
  Constant18/1 -> Product6/1
  [Qac_ref] -> Switch6/3
  Selector3/1 -> Product3/1
  PQreg_On/1 -> AC Voltage Regulator (Vac reg)/3(On), Active Power Regulator (Preg)/3(On), Reactive Power Regulator/5(On)
  Gain3/1 -> DC Voltage Regulator (VDCreg)/1(Vdc_f)
  Constant17/1 -> Switch6/2
  [Vgd_fc] -> AC Voltage Regulator (Vac reg)/2(Vd_f)
  Demux3/2 -> [Vgq_fc]
  Constant16/1 -> Switch5/2
  Reactive Power Regulator/1(Iq_ref) -> Current Regulator (Ireg)/2(Iq_ref)
  Switch5/1 -> DC Voltage Regulator (VDCreg)/2(Vdc_ref)
  [Vgd_fc] -> Reactive Power Regulator/1(Vd_mes)
  PQreg_On1/1 -> Switch1/2, Switch2/2
  Subtract1/1 -> Discrete Mean value2/1
  Product3/1 -> Demux5/1
  Switch2/1 -> PID Controller1/1
  Avoid division by zero5/1 -> Divide2/2
  Step6/1 -> Product6/3
  Demux5/2 -> Subtract1/2
  AC Voltage Regulator (Vac reg)/1(Qac_ref) -> Switch6/1
  Step5/1 -> Product6/2
  Demux/1 -> [Id_fc], Product2/2
  [Pac_ref] -> Active Power Regulator (Preg)/2(Pac_ref)
  [Id_fc] -> Current Regulator (Ireg)/3(Id)
  Second-Order Filter1/1 -> Selector3/1, Product2/1, Demux3/1
  Avoid division by zero1/1 -> Mux/1
  Selector8/1 -> Second-Order Filter2/1
  [Vgd_fc] -> Current Regulator (Ireg)/5(Vd)
  Discrete Mean value2/1 -> Reactive Power Regulator/2(Q_f)
  Vdc_ref/1 -> Switch5/3
  Delay3/1 -> m_dq1/1
  Delay1/1 -> m_dq2/1
  Vs_dq1/1 -> Second-Order Filter1/1
  Iconv_dq1/1 -> Selector8/1
  Demux1/1 -> Switch1/1
  Demux1/2 -> Switch2/1
  Id_dq2/1 -> Demux1/1
  VDCreg_On/1 -> DC Voltage Regulator (VDCreg)/3(On)

== system HVDC_MMC1_EMT/CTRL_DQN1/Subsystem1/AC Voltage Regulator (Vac reg) ==
  note: Active Power Regulator
  Vac_ref : Inport  PortDimensions=1
  Vd_f : Inport  Port=2  PortDimensions=1  SampleTime=Ts
  On : Inport  Port=3  PortDimensions=1  SampleTime=Ts
  Discrete-Time Integrator : DiscreteIntegrator  SampleTime=Ts  LimitOutput=on  UpperSaturationLimit=2  LowerSaturationLimit=-2  ICPrevOutput=DiscIntNeverNeededParam  ICPrevScaledInput=DiscIntNeverNeededParam
  Integrator : Integrator  Commented=on  LimitOutput=on  UpperSaturationLimit=2  LowerSaturationLimit=-2
  Product : Product  RndMeth=Zero
  Product1 : Product  RndMeth=Zero
  Saturation2 : Saturate  UpperLimit=2  LowerLimit=-2  SampleTime=Ts
  Sum : Sum  Inputs=|+-
  Sum6 : Sum  InputSameDT=on  SaturateOnIntegerOverflow=on  SampleTime=Ts  OutDataTypeStr=Inherit: Same as first input
  Switch1 : Switch  Criteria=u2 ~= 0  Threshold=0.5  OutDataTypeStr=double  SaturateOnIntegerOverflow=off  InputSameDT=off
  VdcNom_SM : Constant  SampleTime=Ts
  VdcNom_SM1 : Constant  Value=100  SampleTime=Ts
  Zero-Order Hold : ZeroOrderHold  SampleTime=Ts
  Qac_ref : Outport  SampleTime=Ts  VectorParamsAs1DForOutWhenUnconnected=off
  wires:
  Saturation2/1 -> Qac_ref/1
  Vac_ref/1 -> Switch1/1
  On/1 -> Switch1/2
  Switch1/1 -> Sum/1
  Vd_f/1 -> Switch1/3, Sum/2
  Zero-Order Hold/1 -> Sum6/1
  Discrete-Time Integrator/1 -> Sum6/2
  Sum6/1 -> Saturation2/1
  VdcNom_SM1/1 -> Product/1
  Product1/1 -> Zero-Order Hold/1
  Product/1 -> Discrete-Time Integrator/1
  VdcNom_SM/1 -> Product1/1
  Sum/1 -> Product1/2, Product/2
